simulink model "soc1"  (R2018a)
settings: Solver=VariableStepAuto  StartTime=0.0  StopTime=3000  RelTol=1e-3
libraries: nesl_utility x10, fl_lib x9, simrfV2elements x3, elec_lib x2, powerlib x1
settings Model: Creator=shiekhsoliha  LastModifiedBy=shiekhsoliha

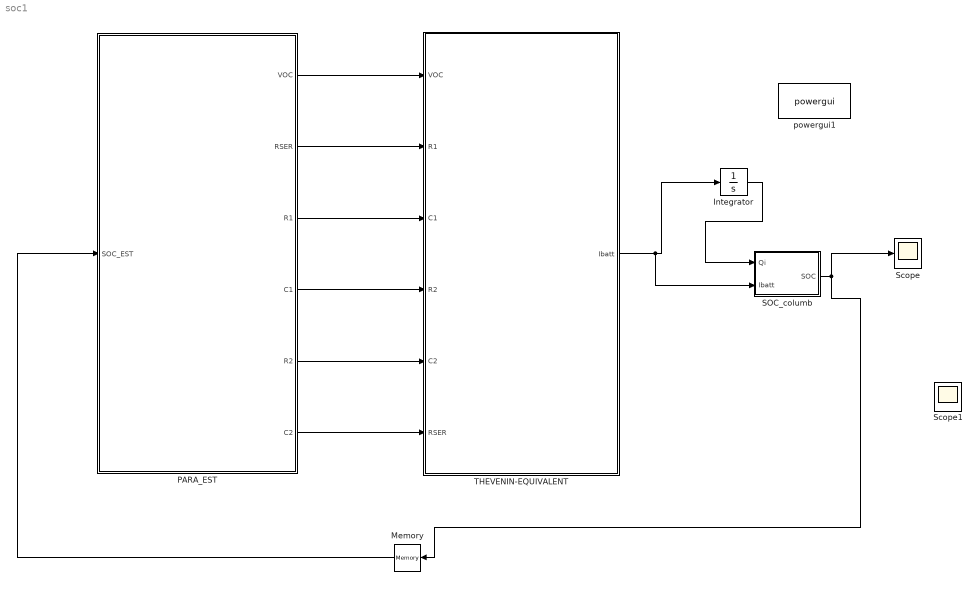
== system soc1 ==
  Integrator : Integrator
  Memory : Memory  InitialCondition=1
  PARA_EST : Subsystem
  SOC_columb : MATLAB Function  TreatAsAtomicUnit=on
  Scope : Scope
  Scope1 : Scope
  THEVENIN-EQUIVALENT : Subsystem
  powergui1 : powerlib/powergui  Priority=1  SimulationMode=Discrete  SampleTime=50e-6  frequency=60  Iterations=50  frequencyindice=60  Pbase=100e6  ErrMax=1e-4  UnitsV=kV  UnitsW=MW  buscounter=0  FunctionMessages=off  echomessages=off  EnableUseOfTLC=off  CurrentSourceSwitches=off  DisableSnubberDevices=off  DisableRonSwitches=off  DisableVfSwitches=off  DisplayEquations=off  SolverType=Tustin/Backward Euler (TBE)  Interpol=off  ExternalGateDelay=off  methode=off  Ts=100  x0status=blocks  SPID=off  SwTol=0  HookPort=off  RestoreLinks=warning  ResistiveCurrentMeasurement=off  Frange=[0:2:500]  Ylog=off  Xlog=on  ShowGrid=off  save=off  variable=ZData  structure=0  ZoomFFT=off  StartTime=0.0  cycles=1  DisplayStyle=1  fundamental=60  FreqAxis=off  MaxFrequency=1000  frequencyindicesteady=1  RmsSteady=1  display=off
  wires:
  PARA_EST/1(VOC) -> THEVENIN-EQUIVALENT/1(VOC)
  PARA_EST/2(RSER) -> THEVENIN-EQUIVALENT/2(R1)
  PARA_EST/3(R1) -> THEVENIN-EQUIVALENT/3(C1)
  PARA_EST/4(C1) -> THEVENIN-EQUIVALENT/4(R2)
  PARA_EST/5(R2) -> THEVENIN-EQUIVALENT/5(C2)
  PARA_EST/6(C2) -> THEVENIN-EQUIVALENT/6(RSER)
  THEVENIN-EQUIVALENT/1(Ibatt) -> SOC_columb/2(Ibatt), Integrator/1
  SOC_columb/1(SOC) -> Memory/1, Scope/1
  Memory/1 -> PARA_EST/1(SOC_EST)
  Integrator/1 -> SOC_columb/1(Qi)

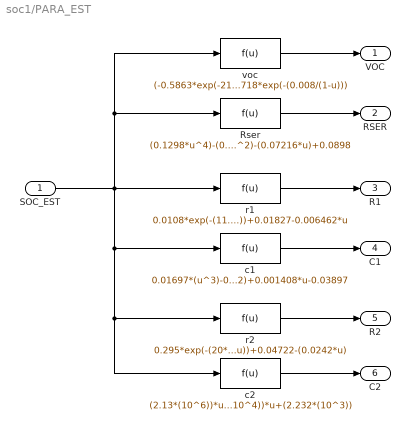
== system soc1/PARA_EST ==
  SOC_EST : Inport
  Rser : Fcn  Expr=(0.1298*u^4)-(0.2892*u^3)+(0.2273*u^2)-(0.07216*u)+0.0898
  c1 : Fcn  Expr=0.01697*(u^3)-0.001007*(u^2)+0.001408*u-0.03897
  c2 : Fcn  Expr=(2.13*(10^6))*u^6-(6.007*(10^6))*(u^5)+(6.271*(10^6))*u^4-(2.958*(10^6))*u^3+(5.998*(10^5))*u^2-(3.102*(10^4))*u+(2.232*(10^3))
  r1 : Fcn  Expr=0.0108*exp(-(11.03*u))+0.01827-0.006462*u
  r2 : Fcn  Expr=0.295*exp(-(20*u))+0.04722-(0.0242*u)
  voc : Fcn  Expr=(-0.5863*exp(-21.90*u))+3.414+0.1102*u-0.1718*exp(-(0.008/(1-u)))
  VOC : Outport
  RSER : Outport  Port=2
  R1 : Outport  Port=3
  C1 : Outport  Port=4
  R2 : Outport  Port=5
  C2 : Outport  Port=6
  wires:
  r1/1 -> R1/1
  c2/1 -> C2/1
  c1/1 -> C1/1
  voc/1 -> VOC/1
  r2/1 -> R2/1
  Rser/1 -> RSER/1
  SOC_EST/1 -> c2/1, r2/1, c1/1, Rser/1, voc/1, r1/1

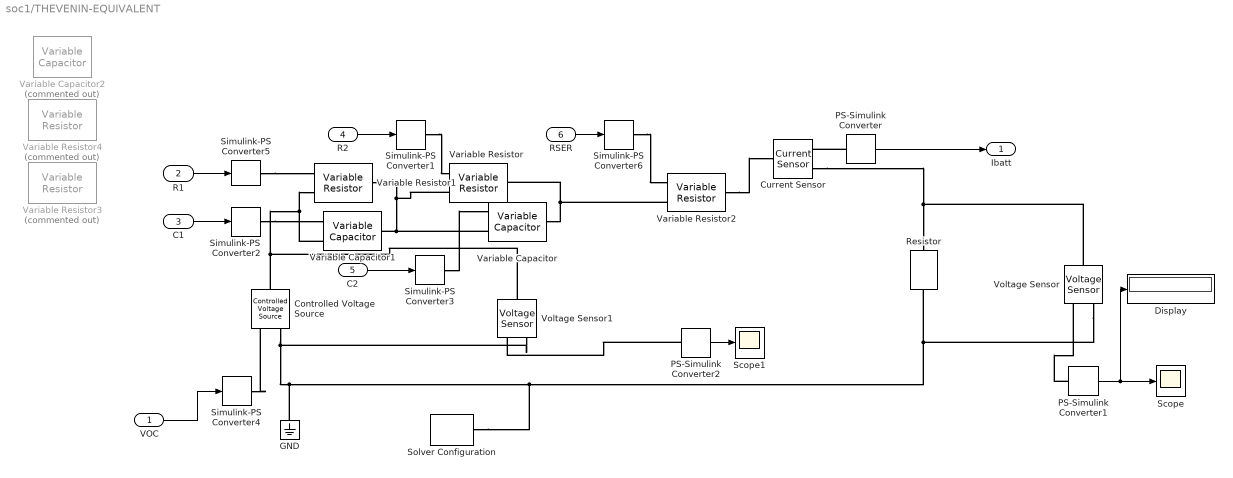
== system soc1/THEVENIN-EQUIVALENT ==
  VOC : Inport
  R1 : Inport  Port=2
  C1 : Inport  Port=3
  R2 : Inport  Port=4
  C2 : Inport  Port=5
  RSER : Inport  Port=6
  Controlled Voltage Source : fl_lib/Electrical/Electrical Sources/Controlled Voltage Source
  Current Sensor : fl_lib/Electrical/Electrical Sensors/Current Sensor
  Display : Display
  GND : fl_lib/Electrical/Electrical Elements/Electrical Reference
  PS-Simulink Converter : nesl_utility/PS-Simulink Converter  PhysicalDomain=network_engine_domain  SubClassName=ps_output  LeftPortType=input  RightPortType=output  PseudoPeriodic=off  Frequencies=[]  Unit=1  AffineConversion=off
  PS-Simulink Converter1 : nesl_utility/PS-Simulink Converter  PhysicalDomain=network_engine_domain  SubClassName=ps_output  LeftPortType=input  RightPortType=output  PseudoPeriodic=off  Frequencies=[]  Unit=1  AffineConversion=off
  PS-Simulink Converter2 : nesl_utility/PS-Simulink Converter  PhysicalDomain=network_engine_domain  SubClassName=ps_output  LeftPortType=input  RightPortType=output  PseudoPeriodic=off  Frequencies=[]  Unit=1  AffineConversion=off
  Resistor : fl_lib/Electrical/Electrical Elements/Resistor  R=10 Ohm  i_specify=off  i_priority=None  i=0 A  i_nominal_specify=off  i_nominal_unit=A  i_nominal_value=1  v_specify=off  v_priority=None  v=0 V  v_nominal_specify=off  v_nominal_unit=V  v_nominal_value=1
  Scope : Scope
  Scope1 : Scope
  Simulink-PS Converter{1..6} (6 alike) : nesl_utility/Simulink-PS Converter  PhysicalDomain=network_engine_domain  SubClassName=ps_input  LeftPortType=input  RightPortType=output  PseudoPeriodic=off  Frequencies=[]  NoiseDistribution=none  NoiseParameters=[]  Unit=1  AffineConversion=off  FilteringAndDerivatives=zero  SimscapeFilterOrder=1  InputFilterTimeConstant=0.001  UdotUserProvided=0
  Solver Configuration : nesl_utility/Solver Configuration  PhysicalDomain=network_engine_domain  SubClassName=solver  LeftPortType=input  RightPortType=generic  Tones=[]  Harmonics=[]  SimulateNoise=off  Profile=off  UseLocalSampling=off  EnableSwitchedLinearOptims=on  FrequencyDomain=off  UseCCode=off  RelTol=0.001  AbsTol=1e-06  MinStep=1e-09  ToWorkspace=off  RevertToSquareIcSolve=off  NumHomotopyIterations=100  PhasorMode=off  PhasorModeNumHarmonics=1  DoDC=off  ResidualTolerance=1e-09  UseLocalSolver=off  LocalSolverChoice=NE_BACKWARD_EULER_ADVANCER  LocalSolverSampleTime=0.001  DoFixedCost=off  MaxNonlinIter=3  MaxModeIter=2  LinearAlgebra=Sparse  EquationFormulation=NE_TIME_EF  DelaysMemoryBudget=1024  AutomaticFiltering=on  FilteringTimeConstant=0.001
  Variable Capacitor2 : simrfV2elements/Variable Capacitor  Commented=on  classname=varcapacitor
      settings: SourceProductName=RF Blockset  SourceProductBaseCode=RB
  Variable Resistor3 : simrfV2elements/Variable Resistor  Commented=on  classname=varresistor  hasNoise=on
      settings: SourceProductName=RF Blockset  SourceProductBaseCode=RB
  Variable Resistor4 : simrfV2elements/Variable Resistor  Commented=on  classname=varresistor  hasNoise=on
      settings: SourceProductName=RF Blockset  SourceProductBaseCode=RB
  Variable Capacitor : elec_lib/Passive Devices/Variable Capacitor  prm=2  Cmin=1e-9 F  r=0 Ohm  v0=0 V  q0=0 C
      settings: SourceProductName=Simscape Electronics  SourceProductBaseCode=SN
  Variable Capacitor1 : elec_lib/Passive Devices/Variable Capacitor  prm=2  Cmin=1e-9 F  r=0 Ohm  v0=0 V  q0=0 C
      settings: SourceProductName=Simscape Electronics  SourceProductBaseCode=SN
  Variable Resistor : fl_lib/Electrical/Electrical Elements/Variable Resistor  Rmin=.00001 Ohm  i_specify=off  i_priority=None  i=0 A  i_nominal_specify=off  i_nominal_unit=A  i_nominal_value=1  v_specify=off  v_priority=None  v=0 V  v_nominal_specify=off  v_nominal_unit=V  v_nominal_value=1
  Variable Resistor1 : fl_lib/Electrical/Electrical Elements/Variable Resistor  Rmin=0 Ohm  i_specify=off  i_priority=None  i=0 A  i_nominal_specify=off  i_nominal_unit=A  i_nominal_value=1  v_specify=off  v_priority=None  v=0 V  v_nominal_specify=off  v_nominal_unit=V  v_nominal_value=1
  Variable Resistor2 : fl_lib/Electrical/Electrical Elements/Variable Resistor  Rmin=0 Ohm  i_specify=off  i_priority=None  i=0 A  i_nominal_specify=off  i_nominal_unit=A  i_nominal_value=1  v_specify=off  v_priority=None  v=0 V  v_nominal_specify=off  v_nominal_unit=V  v_nominal_value=1
  Voltage Sensor : fl_lib/Electrical/Electrical Sensors/Voltage Sensor
  Voltage Sensor1 : fl_lib/Electrical/Electrical Sensors/Voltage Sensor
  Ibatt : Outport
  wires:
  VOC/1 -> Simulink-PS Converter4/1
  R2/1 -> Simulink-PS Converter1/1
  C1/1 -> Simulink-PS Converter2/1
  R1/1 -> Simulink-PS Converter5/1
  C2/1 -> Simulink-PS Converter3/1
  PS-Simulink Converter/1 -> Ibatt/1
  RSER/1 -> Simulink-PS Converter6/1
  PS-Simulink Converter1/1 -> Display/1, Scope/1
  PS-Simulink Converter2/1 -> Scope1/1
  connections:
  Simulink-PS Converter3/RConn1 -- Variable Capacitor/LConn1
  Simulink-PS Converter6/RConn1 -- Variable Resistor2/LConn1
  Simulink-PS Converter5/RConn1 -- Variable Resistor1/LConn1
  Simulink-PS Converter2/RConn1 -- Variable Capacitor1/LConn1
  Simulink-PS Converter1/RConn1 -- Variable Resistor/LConn1
  Simulink-PS Converter4/RConn1 -- Controlled Voltage Source/RConn1
  Variable Resistor2/RConn1 -- Current Sensor/LConn1
  PS-Simulink Converter/LConn1 -- Current Sensor/RConn1
  Current Sensor/RConn2 -- Voltage Sensor/LConn1 -- Resistor/LConn1
  Variable Capacitor1/LConn2 -- Voltage Sensor1/LConn1 -- Controlled Voltage Source/LConn1 -- Variable Resistor1/LConn2
  Variable Resistor1/RConn1 -- Variable Resistor/LConn2 -- Variable Capacitor/LConn2 -- Variable Capacitor1/RConn1
  Variable Capacitor/RConn1 -- Variable Resistor2/LConn2 -- Variable Resistor/RConn1
  Controlled Voltage Source/RConn2 -- Voltage Sensor1/RConn2 -- GND/LConn1 -- Voltage Sensor/RConn2 -- Resistor/RConn1 -- Solver Configuration/RConn1
  PS-Simulink Converter1/LConn1 -- Voltage Sensor/RConn1
  PS-Simulink Converter2/LConn1 -- Voltage Sensor1/RConn1

== matlab function soc1/SOC_columb ==
  data: Qi input; Ibatt input; SOC output
function SOC = fcn(Qi,Ibatt)
SOC_INITIAL=.9;
Qo=4*3600;
pQi=Qi/Qo;
if Ibatt>0
    SOC=SOC_INITIAL-pQi;
else 
    SOC=SOC_INITIAL+pQi;
end
